simulink model "simVINS"  (R2018a)
settings: Solver=FixedStepDiscrete  StartTime=0.0  StopTime=inf  FixedStep=1/Fs  RelTol=1e-3  EnableMultiTasking=on
PreLoadFcn:
  | calibrateSFMA=false
  | modelDef = getModelDef(calibrateSFMA);
  | load VINS_bus_definitions.mat;
  | 
  | imuLocationMm = [6 -4.5 -16.8];
  | dejitter_on = true;
  | fidPosUncert = 0.01;
  | 
  | Fs = 1000;  % nominal IMU sampling rate (Hz)
  | 
  | gyroCalBiases = [0;0;0];
  | gyroCalMatrix = eye(3);
  | gyroGsensMatrix = zeros(3,3);
  | Hgyro = [1 0 0 0; 0 1 0 0; 0 0 1 0];
  | 
  | accelCalBiases = [0;0;0];
  | accelCalMatrix = eye(3);
  | Haccel = [1 0 0 0; 0 1 0 0; 0 0 1 0];
  | 
  | imuPar = getImuPar('lmvpCalibrated');
  | optical_cal = getOpticalCalfile();
  | 
  | lastUsedMgyr = zeros(3,3);
  | 
  | 
  | 
  | simData = true;
  | if simData
  |    load truthTrajectory.mat;
  | 
  |    % set Fs based on the timestamps
  |    Fs = 1/mean(diff(truthTrajectory.t.Data));
  |    if Fs>990
  |      Fs = Fs/2;  % bring 1000 Hz down to 500 Hz for faster simulation
  |    end
  | end
  | 
  | imageTensor = uint8(zeros(384,384,2));
  | imageTstamps = 0;
  | useImages = false;
  | useFeatures = false;
  | imageFeatureMatrix = zeros(10,263);
  | 
  | bundle_num_points = 400;
  | bundle_num_frames = 60;
  | 
  | % get rid of following lines if no longer using global data stores to send truth data into VINS
  | truthTraj = Simulink.Signal;
  | truthTraj.DataType = 'Bus: truthTrajectoryBus';
  | truthTraj.InitialValue = '0';
  | truthTraj.Complexity = 'Real';
StartFcn:
  | cd 'C:\Users\efoxlin\Documents\MATLAB\VINS';
undefined symbols (not defined in the file or in its folder): accels, gyros, jumpToXyz, jumpToYaw, tstamp_imu_us, tstamp_vidcap_us, xyz, yaw
libraries: simulink x6, dspmtrx3 x6, dspsrcs4 x6, vrlib x5, dspsigops x2, dspstat3 x2, realtime_pacer_lib x1, dspswit3 x1
(part 2 of 2)

== system simVINS/simulatedData/simulateIdealImuWithOffset/centripetalTangential ==
  Cbn : Inport
  ain : Inport  Port=2
  w : Inport  Port=3
  wdot : Inport  Port=4
  r : Inport  Port=5
  Cross Product : vrlib/Utilities/Cross Product
      settings: SourceProductBaseCode=VR
  Cross Product1 : vrlib/Utilities/Cross Product
      settings: SourceProductBaseCode=VR
  Cross Product2 : vrlib/Utilities/Cross Product
      settings: SourceProductBaseCode=VR
  Matrix Multiply : Product  Multiplication=Matrix(*)
  Sum : Sum  Inputs=|++
  Sum1 : Sum  Inputs=|++
  aout : Outport
  wires:
  w/1 -> Cross Product/1, Cross Product1/1
  r/1 -> Cross Product2/2, Cross Product/2
  Cross Product/1 -> Cross Product1/2
  wdot/1 -> Cross Product2/1
  Sum1/1 -> aout/1
  Cross Product1/1 -> Sum/1
  Cross Product2/1 -> Sum/2
  Cbn/1 -> Matrix Multiply/1
  Sum/1 -> Matrix Multiply/2
  Matrix Multiply/1 -> Sum1/2
  ain/1 -> Sum1/1

== system simVINS/simulatedData/simulateImuErrors/calcDt ==
  t : Inport
  Constant : Constant  Value=0
  Constant10 : Constant
  Difference : simulink/Discrete/Difference  ICPrevInput=0.0  OutMin=[]  OutMax=[]  OutDataType=fixdt(1, 16)  OutScaling=2^-10  DoSatur=off
  Switch : Switch  Criteria=u2 > Threshold
  Unit Delay : UnitDelay  SampleTime=-1
  Dt : Outport
  wires:
  Unit Delay/1 -> Switch/2
  Constant/1 -> Switch/3
  Switch/1 -> Dt/1
  Difference/1 -> Switch/1
  t/1 -> Difference/1
  Constant10/1 -> Unit Delay/1

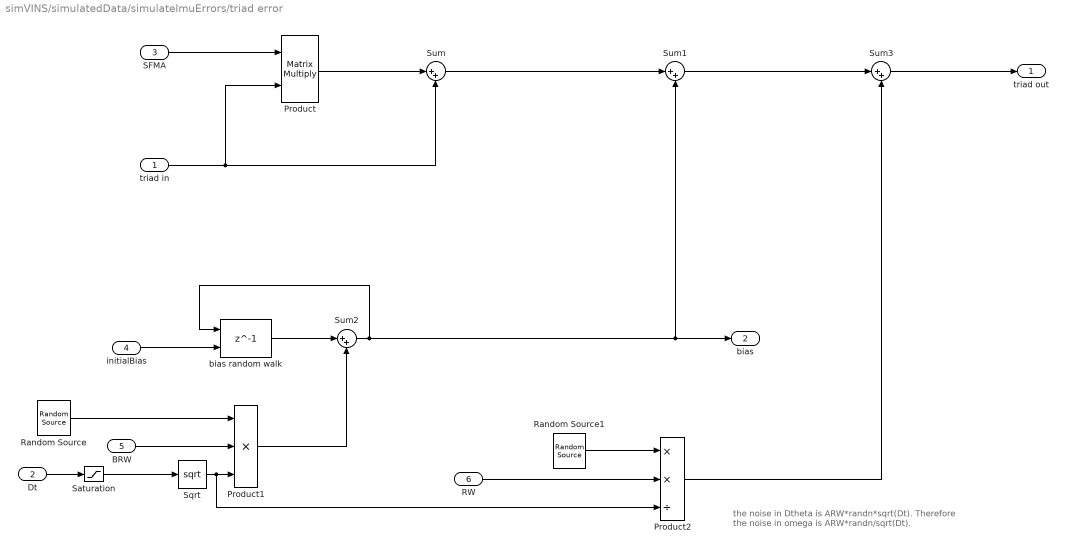
== system simVINS/simulatedData/simulateImuErrors/triad error ==
  note: the noise in Dtheta is ARW*randn*sqrt(Dt). Therefore the noise in omega is ARW*randn/sqrt(Dt).
  triad in : Inport
  Dt : Inport  Port=2
  SFMA : Inport  Port=3
  initialBias : Inport  Port=4
  BRW : Inport  Port=5
  RW : Inport  Port=6
  Product : Product  Multiplication=Matrix(*)
  Product1 : Product  Inputs=3
  Product2 : Product  Inputs=**/
  Random Source : dspsrcs4/Random Source  SrcType=Gaussian  NormMethod=Ziggurat  CltLength=12  MinVal=0  MaxVal=1  MeanVal=[0;0;0]  VarVal=1  RepMode=Not repeatable  rawSeed=1  IsInherit=off  SampMode=Discrete  SampTime=1/Fs  SampFrame=1  DataType=Double  OutComplex=Real  OutputFrames=off
  Random Source1 : dspsrcs4/Random Source  SrcType=Gaussian  NormMethod=Ziggurat  CltLength=12  MinVal=0  MaxVal=1  MeanVal=[0;0;0]  VarVal=1  RepMode=Not repeatable  rawSeed=1  IsInherit=off  SampMode=Discrete  SampTime=1/Fs  SampFrame=1  DataType=Double  OutComplex=Real  OutputFrames=off
  Saturation : Saturate  LowerLimit=0.0005
  Sqrt : Sqrt  SaturateOnIntegerOverflow=on
  Sum{,1..3} (4 alike) : Sum  Inputs=|++
  bias random walk : Delay  DelayLength=1  InitialConditionSource=Input port
      settings: InputPortMap=u0,p4
  triad out : Outport
  bias : Outport  Port=2
  wires:
  triad in/1 -> Sum/2, Product/2
  SFMA/1 -> Product/1
  Product/1 -> Sum/1
  Sum/1 -> Sum1/1
  Sum1/1 -> Sum3/1
  initialBias/1 -> bias random walk/2
  bias random walk/1 -> Sum2/1
  Sum2/1 -> bias/1, Sum1/2, bias random walk/1
  Dt/1 -> Saturation/1
  Sqrt/1 -> Product2/3, Product1/3
  BRW/1 -> Product1/2
  Product1/1 -> Sum2/2
  RW/1 -> Product2/2
  Sum3/1 -> triad out/1
  Product2/1 -> Sum3/2
  Random Source/1 -> Product1/1
  Random Source1/1 -> Product2/1
  Saturation/1 -> Sqrt/1

== system simVINS/simulatedData/simulateImuErrors/triad error1 ==
  note: the noise in Dtheta is ARW*randn*sqrt(Dt). Therefore the noise in omega is ARW*randn/sqrt(Dt).
  triad in : Inport
  Dt : Inport  Port=2
  SFMA : Inport  Port=3
  initialBias : Inport  Port=4
  BRW : Inport  Port=5
  RW : Inport  Port=6
  Product : Product  Multiplication=Matrix(*)
  Product1 : Product  Inputs=3
  Product2 : Product  Inputs=**/
  Random Source : dspsrcs4/Random Source  SrcType=Gaussian  NormMethod=Ziggurat  CltLength=12  MinVal=0  MaxVal=1  MeanVal=[0;0;0]  VarVal=1  RepMode=Not repeatable  rawSeed=1  IsInherit=off  SampMode=Discrete  SampTime=1/Fs  SampFrame=1  DataType=Double  OutComplex=Real  OutputFrames=off
  Random Source1 : dspsrcs4/Random Source  SrcType=Gaussian  NormMethod=Ziggurat  CltLength=12  MinVal=0  MaxVal=1  MeanVal=[0;0;0]  VarVal=1  RepMode=Not repeatable  rawSeed=1  IsInherit=off  SampMode=Discrete  SampTime=1/Fs  SampFrame=1  DataType=Double  OutComplex=Real  OutputFrames=off
  Saturation : Saturate  LowerLimit=0.0005
  Sqrt : Sqrt  SaturateOnIntegerOverflow=on
  Sum{,1..3} (4 alike) : Sum  Inputs=|++
  bias random walk : Delay  DelayLength=1  InitialConditionSource=Input port
      settings: InputPortMap=u0,p4
  triad out : Outport
  bias : Outport  Port=2
  wires:
  triad in/1 -> Sum/2, Product/2
  SFMA/1 -> Product/1
  Product/1 -> Sum/1
  Sum/1 -> Sum1/1
  Sum1/1 -> Sum3/1
  initialBias/1 -> bias random walk/2
  bias random walk/1 -> Sum2/1
  Sum2/1 -> bias/1, Sum1/2, bias random walk/1
  Dt/1 -> Saturation/1
  Sqrt/1 -> Product2/3, Product1/3
  BRW/1 -> Product1/2
  Product1/1 -> Sum2/2
  RW/1 -> Product2/2
  Sum3/1 -> triad out/1
  Product2/1 -> Sum3/2
  Random Source/1 -> Product1/1
  Random Source1/1 -> Product2/1
  Saturation/1 -> Sqrt/1

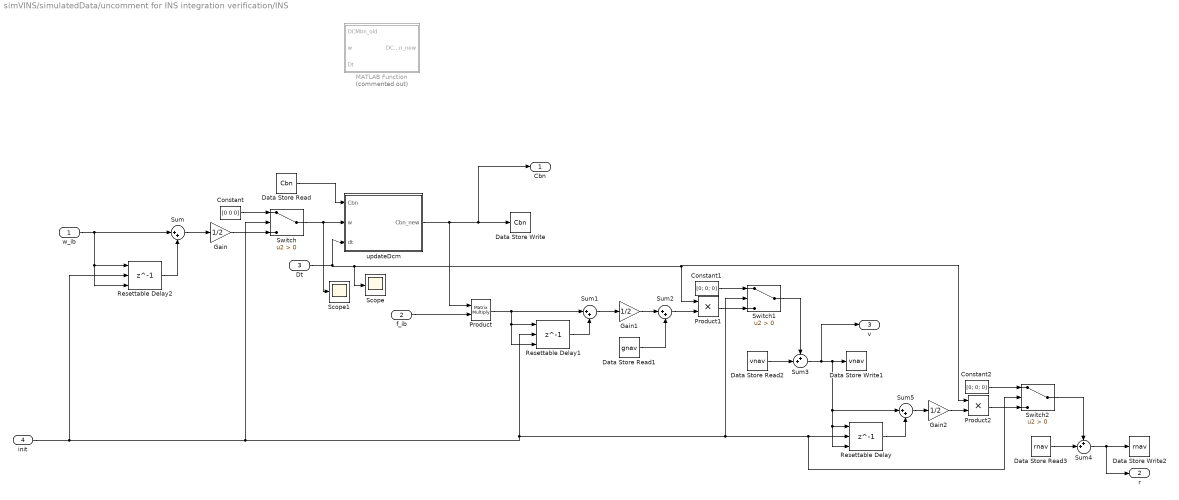
== system simVINS/simulatedData/uncomment for INS integration verification/INS ==
  w_ib : Inport
  f_ib : Inport  Port=2
  Dt : Inport  Port=3
  init : Inport  Port=4
  Constant : Constant  Value=[0 0 0]
  Constant1 : Constant  Value=[0; 0; 0]  VectorParams1D=off
  Constant2 : Constant  Value=[0; 0; 0]  VectorParams1D=off
  Data Store Read : DataStoreRead  DataStoreName=Cbn
  Data Store Read1 : DataStoreRead  DataStoreName=gnav
  Data Store Read2 : DataStoreRead  DataStoreName=vnav
  Data Store Read3 : DataStoreRead  DataStoreName=rnav
  Data Store Write : DataStoreWrite  DataStoreName=Cbn
  Data Store Write1 : DataStoreWrite  DataStoreName=vnav
  Data Store Write2 : DataStoreWrite  DataStoreName=rnav
  Gain : Gain  Gain=1/2
  Gain1 : Gain  Gain=1/2
  Gain2 : Gain  Gain=1/2
  MATLAB Function : MATLAB Function  Commented=on  TreatAsAtomicUnit=on
  Product : Product  Multiplication=Matrix(*)
  Product1 : Product
  Product2 : Product
  Resettable Delay : Delay  DelayLength=1  InitialConditionSource=Input port  ExternalReset=Level hold
      settings: InputPortMap=u0,r5,p4
  Resettable Delay1 : Delay  DelayLength=1  InitialConditionSource=Input port  ExternalReset=Level hold
      settings: InputPortMap=u0,r5,p4
  Resettable Delay2 : Delay  DelayLength=1  InitialConditionSource=Input port  ExternalReset=Level hold
      settings: InputPortMap=u0,r5,p4
  Scope : Scope
  Scope1 : Scope
  Sum{,1..2,5} (4 alike) : Sum  Inputs=|++
  Sum3 : Sum  Inputs=++|
  Sum4 : Sum  Inputs=++|
  Switch : Switch  Criteria=u2 > Threshold
  Switch1 : Switch  Criteria=u2 > Threshold
  Switch2 : Switch  Criteria=u2 > Threshold
  updateDcm : MATLAB Function  TreatAsAtomicUnit=on
  Cbn : Outport
  r : Outport  Port=2
  v : Outport  Port=3
  wires:
  Resettable Delay1/1 -> Sum1/2
  Resettable Delay/1 -> Sum5/2
  Gain2/1 -> Product2/2
  Sum3/1 -> v/1, Data Store Write1/1, Sum5/1, Resettable Delay/1, Resettable Delay/3
  Sum5/1 -> Gain2/1
  Sum4/1 -> r/1, Data Store Write2/1
  Data Store Read3/1 -> Sum4/2
  Switch1/1 -> Sum3/1
  Data Store Read2/1 -> Sum3/2
  Gain1/1 -> Sum2/1
  Sum1/1 -> Gain1/1
  Product/1 -> Sum1/1, Resettable Delay1/1, Resettable Delay1/3
  Sum2/1 -> Product1/2
  Data Store Read1/1 -> Sum2/2
  f_ib/1 -> Product/2
  Sum/1 -> Gain/1
  Resettable Delay2/1 -> Sum/2
  updateDcm/1(Cbn_new) -> Cbn/1, Data Store Write/1, Product/1
  w_ib/1 -> Sum/1, Resettable Delay2/3, Resettable Delay2/1
  Dt/1 -> updateDcm/3(dt), Scope/1, Product1/1, Product2/1
  init/1 -> Resettable Delay2/2, Switch/2, Switch1/2, Switch2/2, Resettable Delay/2, Resettable Delay1/2
  Data Store Read/1 -> updateDcm/1(Cbn)
  Gain/1 -> Switch/3
  Constant/1 -> Switch/1
  Product1/1 -> Switch1/3
  Constant1/1 -> Switch1/1
  Product2/1 -> Switch2/3
  Switch2/1 -> Sum4/1
  Constant2/1 -> Switch2/1
  Switch/1 -> updateDcm/2(w), Scope1/1

== system simVINS/simulatedData/uncomment for INS integration verification/calcDt ==
  t : Inport
  Constant : Constant  Value=0
  Constant10 : Constant
  Difference : simulink/Discrete/Difference  ICPrevInput=0.0  OutMin=[]  OutMax=[]  OutDataType=fixdt(1, 16)  OutScaling=2^-10  DoSatur=off
  Switch : Switch  Criteria=u2 > Threshold
  Unit Delay : UnitDelay  SampleTime=-1
  Dt : Outport
  wires:
  Constant10/1 -> Unit Delay/1
  t/1 -> Difference/1
  Difference/1 -> Switch/1
  Switch/1 -> Dt/1
  Constant/1 -> Switch/3
  Unit Delay/1 -> Switch/2

== system simVINS/simulatedData/uncomment for INS integration verification/setInitialInsStates ==
  rnav : Inport
  vnav : Inport  Port=2
  Cbn : Inport  Port=3
  omega : Inport  Port=4
  Enable : EnablePort  ShowOutputPort=on
  Constant : Constant  Value=imuLocationMm/1000
  Cross Product : vrlib/Utilities/Cross Product
      settings: SourceProductBaseCode=VR
  Data Store Write2 : DataStoreWrite  DataStoreName=vnav
  Data Store Write3 : DataStoreWrite  DataStoreName=rnav
  Data Store Write8 : DataStoreWrite  DataStoreName=Cbn
  Gain : Gain  Gain=-1
  Matrix Multiply : Product  Multiplication=Matrix(*)
  Matrix Multiply1 : Product  Multiplication=Matrix(*)
  Sum : Sum  Inputs=++|
  Sum1 : Sum  Inputs=++|
  Out1 : Outport  OutputWhenDisabled=reset  InitialOutput=false
  wires:
  Enable/1 -> Out1/1
  rnav/1 -> Sum/2
  Cbn/1 -> Matrix Multiply1/1, Matrix Multiply/1, Data Store Write8/1
  Constant/1 -> Gain/1, Matrix Multiply/2
  Matrix Multiply/1 -> Sum/1
  Sum/1 -> Data Store Write3/1
  vnav/1 -> Sum1/2
  Sum1/1 -> Data Store Write2/1  "velocity at imu"
  omega/1 -> Cross Product/1
  Cross Product/1 -> Matrix Multiply1/2
  Matrix Multiply1/1 -> Sum1/1
  Gain/1 -> Cross Product/2

== matlab function simVINS/simulatedData/uncomment for INS integration verification/INS/updateDcm ==
  data: Cbn input; Cbn_new output; w input; dt input
function Cbn_new = update_dcm(Cbn, w, dt)

% Update attitude according to TW p.312 approximated to sixth order

rot=w*dt;
rot_norm=norm(rot);
sr_a=1-(rot_norm^2/6)+(rot_norm^4/120);
sr_b=(1/2)-(rot_norm^2/24)+(rot_norm^4/720);
mx_a=eye(3)+sr_a*skew(rot)+sr_b*skew(rot)*skew(rot);

Cbn_new=Cbn*mx_a;


function res=skew(inp_vr)
res=[0 			-inp_vr(3)	inp_vr(2); ...
     inp_vr(3)	0			-inp_vr(1);...
	 -inp_vr(2)	inp_vr(1)	0];

== matlab function simVINS/simulatedData/reportOutputs/MATLAB Function3 ==
  data: Cbn input; eul output size=[3,1]
function eul = dcm2euler(Cbn)

%DCM is Cbn (transforms vectors from b to n)
%eul defined as zyx sequence (yaw,pitch,roll),  but listed in
%roll,pitch,yaw order


pitch=asin(-Cbn(3,1));  %pitch is assumed to be [-pi pi]. singular at pi. use ad-hoc methods to remedy this deficiency
roll=atan2(Cbn(3,2), Cbn(3,3));
heading = atan2(Cbn(2,1), Cbn(1,1));
eul=[roll;pitch;heading];

== matlab function simVINS/simulatedData/uncomment for INS integration verification/MATLAB Function3 ==
  data: Cbn input; eul output size=[3,1]
function eul = dcm2euler(Cbn)

%DCM is Cbn (transforms vectors from b to n)
%eul defined as zyx sequence (yaw,pitch,roll),  but listed in
%roll,pitch,yaw order


pitch=asin(-Cbn(3,1));  %pitch is assumed to be [-pi pi]. singular at pi. use ad-hoc methods to remedy this deficiency
roll=atan2(Cbn(3,2), Cbn(3,3));
heading = atan2(Cbn(2,1), Cbn(1,1));
eul=[roll;pitch;heading];

== matlab function simVINS/simulatedData/uncomment for INS integration verification/INS/MATLAB Function ==
  data: DCMbn_old input; DCMbn_new output; w input; Dt input
function DCMbn_new  = bodupdat(DCMbn_old, w, Dt)
%BODUPDAT		Update the direction cosine matrix
%              for body motion (relative to inertial space).
%              The function is thus acting upon the strapdown
%              gyro outputs.
%       
%	DCMbn_new = bodupdat(DCMbn_old,ang_vect)
%     or
%  [DCMbn_new,DCMbb] = bodupdat(DCMbn_old,ang_vect)
%
%   INPUTS
%       DCMbn_old  = current direction cosine matrix providing the
%                    transformation from body to nav coordinates
%
%       ang_vect = incremental integral of body angular
%                  rate vector; in the absence of coning
%                  (i.e., angular rate vector is constant
%                  over the integration interval), this
%                  is the output of the rate-integrating
%                  gyros.
%          ang_vect(1) = x-component (roll);
%          ang_vect(2) = y-component (pitch);
%          ang_vect(3) = z-component (yaw);
%
%   OUTPUTS
%       DCMbn_new = updated direction cosine matrix relating the
%                   current body-frame to the previous
%                   navigation-frame.  Note that the update of
%                   the navigation frame (which is related to
%                   the local-level frame) is accomplished in
%                   function LCLEVUPD
%
%       DCMbb = direction cosine matrix providing the
%               transformation from the body coordinates at
%               time k+1 to the body coordinates at time k
%

%	M. & S. Braasch 4-98
%	Copyright (c) 1997-98 by GPSoft LLC
%	All Rights Reserved.
%

if nargin<3,error('insufficient number of input arguments'),end
ang_vect = w*Dt;

S = skewsymm(ang_vect);
magn = norm(ang_vect);
if magn == 0
   DCMbb = eye(3);
else
   DCMbb = eye(3) + (sin(magn)/magn)*S + ( (1-cos(magn))/magn^2 )*S*S;
end
DCMbn_new = DCMbn_old*DCMbb;

== matlab function simVINS/readFromFile/fetchImages/MATLAB Function ==
  data: imgNum input; left output; right output; imageTensor input
function [left, right] = getImg(imgNum, imageTensor)

left = imageTensor(:,:,1, imgNum);
right = imageTensor(:,:,2, imgNum);

== matlab function simVINS/readFromFile/printTime/MATLAB Function ==
  data: u input
function  printTime(u)
%#codegen

% using fileId = 1  only generates a printf in the generated code
% fileId = 2 also causes prints in the matlab console

fprintf(1, "\r %f", u);

== matlab function simVINS/readFromFile/fetchFeatures/MATLAB Function ==
  data: nPoints output; IDs output size=[400 1]; imgNum input; leftPts output size=[400, 2]; rightPts output size=[400 2]; imageFeatureMatrix input; xyz output
function [nPoints, IDs, leftPts, rightPts, xyz] = getFeatures(imgNum, imageFeatureMatrix)

nPoints = imageFeatureMatrix(imgNum, 3);

row = imageFeatureMatrix(imgNum, 4:end);
rowNumPts = length(row)/26;  % the first three elements are 1, tstamp, nPts,  followed by 26 values for each point
%// 1, timestamp, # features, REPEATS: {Id, Age, u left (px), v left (px), u right (px), v right (px), x (m), y (m), z (m), isMatched, ORB 1-8 left, ORB 1-8 right}

data = zeros(400, 26);
data(1:rowNumPts, 1:26) = reshape(row, 26, rowNumPts)'; 

IDs = data(:, 1);
leftPts = data(:, 3:4);
rightPts = data(:, 5:6);
xyz = data(:,7:9);

== matlab function simVINS/simVisionSystem/skew ==
  data: inp_vr input; res output
function res=skew(inp_vr)
res=[0 			-inp_vr(3)	inp_vr(2); ...
     inp_vr(3)	0			-inp_vr(1);...
	 -inp_vr(2)	inp_vr(1)	0];

== matlab function simVINS/simulatedData/reportOutputs/MATLAB Function1 ==
  data: Cbn input; quat output size=[4,1]
function quat=dcm2quat(Cbn)

%dcm (Cba) to quaternion (qba)
%Cba:B to A transformation matrix
%qba:B to A quaternion

%Implementation of savage(3-47)


tr=Cbn(1,1)+Cbn(2,2)+Cbn(3,3);
Pa=1+tr;
Pb=1+2*Cbn(1,1)-tr;
Pc=1+2*Cbn(2,2)-tr;
Pd=1+2*Cbn(3,3)-tr;

quat=zeros(4,1);
if (Pa>=Pb && Pa>=Pc && Pa>=Pd)
    quat(1)=0.5*sqrt(Pa);
    quat(2)=(Cbn(3,2)-Cbn(2,3))/4/quat(1);
    quat(3)=(Cbn(1,3)-Cbn(3,1))/4/quat(1);
    quat(4)=(Cbn(2,1)-Cbn(1,2))/4/quat(1);
elseif (Pb>=Pc && Pb>=Pd)
    quat(2)=0.5*sqrt(Pb);
    quat(3)=(Cbn(2,1)+Cbn(1,2))/4/quat(2);
    quat(4)=(Cbn(1,3)+Cbn(3,1))/4/quat(2);
    quat(1)=(Cbn(3,2)-Cbn(2,3))/4/quat(2);
elseif (Pc>=Pd)
    quat(3)=0.5*sqrt(Pc);
    quat(4)=(Cbn(3,2)+Cbn(2,3))/4/quat(3);
    quat(1)=(Cbn(1,3)-Cbn(3,1))/4/quat(3);
    quat(2)=(Cbn(2,1)+Cbn(1,2))/4/quat(3);
else
    quat(4)=0.5*sqrt(Pd);
    quat(1)=(Cbn(2,1)-Cbn(1,2))/4/quat(4);
    quat(2)=(Cbn(1,3)+Cbn(3,1))/4/quat(4);
    quat(3)=(Cbn(3,2)+Cbn(2,3))/4/quat(4);
end

if (quat(1)<=0)
    quat=-quat;
end

== matlab function simVINS/readFromFile/displayPoints ==
  data: Cbn input; r_nb_n input; X input
function  displayPoints(Cbn, r_nb_n, X)

maxpts = 400;

persistent h

if isempty(h)
    figure(100);
    set(gcf,'Renderer','OpenGL');
    x = zeros(1, maxpts); y = zeros(1, maxpts);
    h = plot(x,y,'.'); %,'MarkerSize',2,'MarkerFaceColor','b');
    set(h,'EraseMode','normal');
    xlim([-1.5,1.5]);
    ylim([-1.5,1.5]);
end

nvalid = sum(X(4,:)==1);
if nvalid>3
    
    xyz_n = X(1:3, X(4,:)==1);
    
    xyz_b = Cbn' * (xyz_n - repmat(r_nb_n, 1 , size(xyz_n,2)));
    
    mask = xyz_b(2,:) >= 0.05; %points in front of camera
    u = -xyz_b(1,mask)./xyz_b(2,mask);
    v = xyz_b(3,mask)./xyz_b(2,mask);
    
    x = zeros(1, maxpts); y = zeros(1, maxpts);
    npts = min(maxpts, length(u));
    x(1,1:npts) = u(1,1:npts);
    y(1,1:npts) = -v(1,1:npts);
    
    set(h,'XData',x, 'YData', y);
    drawnow;

end
